simulink model "uzunolan"  (R2020a)
settings: Solver=VariableStepAuto  StartTime=0.0  StopTime=10.0  RelTol=1e-3
PreLoadFcn:
  | Kp=0.35;
  | l = 0.75;
  | g = 9.81;
  | Kc = 2;
  | f = 2;
settings Model: Creator=muham  LastModifiedBy=muham

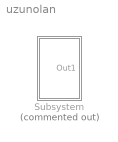
== system uzunolan ==
  Subsystem : Subsystem  Commented=on

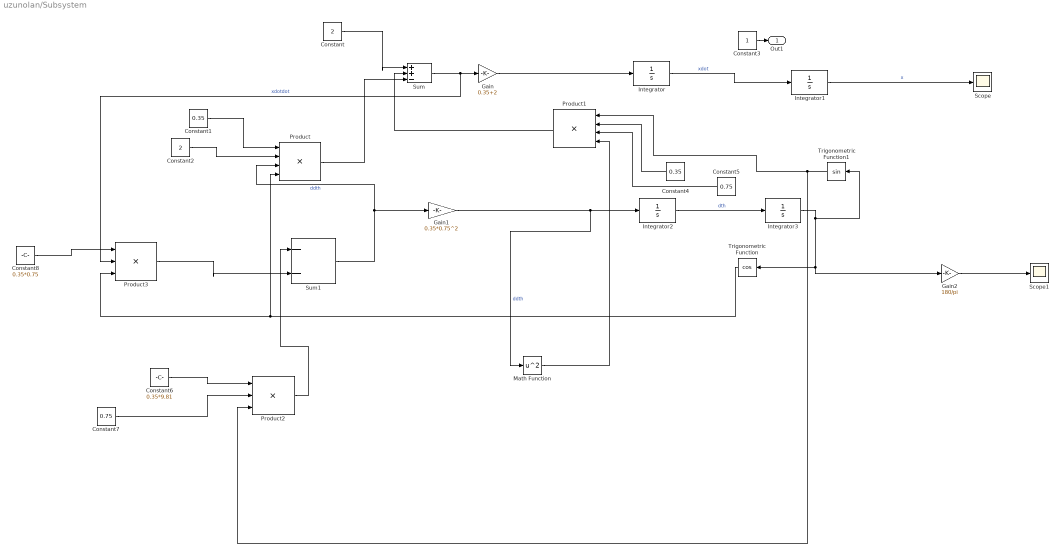
== system uzunolan/Subsystem ==
  Constant : Constant  Value=2
  Constant1 : Constant  Value=0.35
  Constant2 : Constant  Value=2
  Constant3 : Constant
  Constant4 : Constant  Value=0.35
  Constant5 : Constant  Value=0.75
  Constant6 : Constant  Value=0.35*9.81
  Constant7 : Constant  Value=0.75
  Constant8 : Constant  Value=0.35*0.75
  Gain : Gain  Gain=0.35+2
  Gain1 : Gain  Gain=0.35*0.75^2
  Gain2 : Gain  Gain=180/pi
  Integrator : Integrator
  Integrator1 : Integrator  InitialCondition=0.15
  Integrator2 : Integrator
  Integrator3 : Integrator  InitialCondition=pi/3
  Math Function : Math  Operator=square  SaturateOnIntegerOverflow=on
  Product : Product  Inputs=4
  Product1 : Product  Inputs=4
  Product2 : Product  Inputs=3
  Product3 : Product  Inputs=3
  Scope : Scope
  Scope1 : Scope
  Sum : Sum  Inputs=|++-
  Sum1 : Sum  Inputs=|--
  Trigonometric Function : Trigonometry  Operator=cos
  Trigonometric Function1 : Trigonometry
  Out1 : Outport
  wires:
  Trigonometric Function1/1 -> Product2/3, Product1/1
  Gain/1 -> Integrator/1
  Integrator3/1 -> Trigonometric Function1/1, Gain2/1, Trigonometric Function/1
  Gain1/1 -> Math Function/1, Integrator2/1  "ddth"
  Constant6/1 -> Product2/1
  Integrator/1 -> Integrator1/1  "xdot"
  Trigonometric Function/1 -> Product3/3, Product/4
  Constant4/1 -> Product1/2
  Constant7/1 -> Product2/2
  Sum1/1 -> Product/3, Gain1/1  "ddth"
  Integrator2/1 -> Integrator3/1  "dth"
  Product2/1 -> Sum1/1
  Constant3/1 -> Out1/1
  Constant2/1 -> Product/2
  Constant1/1 -> Product/1
  Sum/1 -> Product3/2, Gain/1  "xdotdot"
  Gain2/1 -> Scope1/1
  Product3/1 -> Sum1/2
  Constant8/1 -> Product3/1
  Constant5/1 -> Product1/3
  Constant/1 -> Sum/1
  Product/1 -> Sum/3
  Product1/1 -> Sum/2
  Math Function/1 -> Product1/4
  Integrator1/1 -> Scope/1  "x"
